simulink model "longitudinal_autopilot"  (Simulink 7.7)
settings: Solver=ode45  StartTime=0.0  StopTime=10.0  RelTol=1e-3
settings Model: Creator=mdpratt  LastModifiedBy=mdpratt

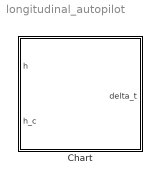
== system longitudinal_autopilot ==
  Chart : Stateflow chart  TreatAsAtomicUnit=on

== stateflow chart Chart ==
  state Climb zone
    during: delta_t =1;
  state Altitude hold zone
  state Descend zone
    during: delta_t = 0;
  Climb zone -> Altitude hold zone : [h >= h_c - delta_h_bar]
  (default) -> Climb zone
  Altitude hold zone -> Climb zone [order 1] : [h < h_c - delta_h_bar]
  Altitude hold zone -> Descend zone [order 2] : [h >= h_c + delta_h_bar]
  Descend zone -> Altitude hold zone : [h < h_c + delta_h_bar]
  data: h input double; h_c input double; delta_t output double
